simulink model "VU_testBtTxRx"  (Simulink 7.5)
settings: Solver=FixedStepDiscrete  SolverMode=SingleTasking  StartTime=0.0  StopTime=inf  FixedStep=0.1  RelTol=1e-3
libraries: lego_nxt_lib x5
settings Model: Creator=jpeytonj  LastModifiedBy=jpeytonj
settings RTWCC: SystemTargetFile=lrt.tlc  GenCodeOnly=on  TemplateMakefile=lrt_ecrobot.tmf  Description=Lego NXT Real-Time Target  ProcessScript=lrt_make_rtw_hook
settings STFCustomTargetCC: ModelReferenceCompliant=off  GeneratePreprocessorConditionals=Disable all  MatFileLogging=on  SystemTargetFile=lrt.tlc
settings GRTTargetCC: ModelReferenceCompliant=off  ParMdlRefBuildCompliant=off  CompOptLevelCompliant=off  ExtModeMexFile=noextcomm
settings CustomProperty: DataType=RTWOptions_EnumType_C__RTtools_VU-LRT_lrt_1codeGenType  Value=Integer-only
settings EnumStrPairs: String=Integer-only

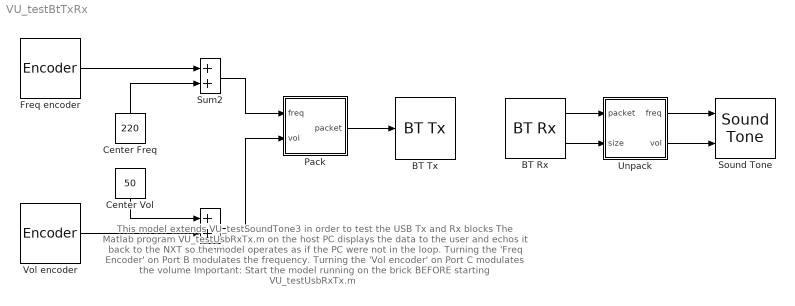
== system VU_testBtTxRx ==
  note: This model extends VU_testSoundTone3 in order to test the USB Tx and Rx blocks
      | The Matlab program VU_testUsbRxTx.m on the host PC displays the data to the user
      | and echos it back to the NXT so the model operates as if the PC were not in the loop.
      | Turning the 'Freq Encoder' on Port B modulates the frequency.
      | Turning the 'Vol encoder' on Port C modulates the volume
      |
      | Important:  Start the model running on the brick BEFORE starting VU_testUsbRxTx.m
  BT Rx : lego_nxt_lib/BT Rx  init_y0=zeros(32,1,'uint8')  mos=Slave  ip=0  st=0.1
  BT Tx : lego_nxt_lib/BT Tx  mos=Slave  ip=0
  Center Freq : Constant  Value=220  OutDataType=fixdt(1, 16)  OutScaling=2^0
  Center Vol : Constant  Value=50  OutDataType=fixdt(1, 16)  OutScaling=2^0
  Freq encoder : lego_nxt_lib/Encoder  port=Port B  st=0.1
  Pack : Stateflow chart  TreatAsAtomicUnit=on
  Sound Tone : lego_nxt_lib/Sound Tone  SystemSampleTime=-1  freqsrc=External  freq=220  volsrc=External  vol=70
  Sum1 : Sum  OutDataTypeMode=uint8  OutDataType=fixdt(1, 16)  OutScaling=2^0  OutDataTypeStr=uint8
  Sum2 : Sum  OutDataTypeMode=uint32  OutDataType=fixdt(1, 16)  OutScaling=2^0  OutDataTypeStr=uint32
  Unpack : Stateflow chart  TreatAsAtomicUnit=on
  Vol encoder : lego_nxt_lib/Encoder  port=Port C  st=0.1
  wires:
  Freq encoder/1 -> Sum2/1
  Center Freq/1 -> Sum2/2
  Vol encoder/1 -> Sum1/2
  Center Vol/1 -> Sum1/1
  BT Rx/1 -> Unpack/1(packet)
  BT Rx/2 -> Unpack/2(size)
  Unpack/1(freq) -> Sound Tone/1
  Sum2/1 -> Pack/1(freq)
  Sum1/1 -> Pack/2(vol)
  Pack/1(packet) -> BT Tx/1
  Unpack/2(vol) -> Sound Tone/2

== matlab function Pack ==
  data: freq input double; packet output double; vol input double
function packet = pack(freq,vol)

%First define the size of the packet
%using nullcopy to avoid generating unnecessary code
%uint32(freq)=4Bytes;  uint8(vol)=1Byte
packet= eml.nullcopy(zeros(5,1,'uint8'));

%Now construct the packet
packet= [typecast(freq,'uint8') typecast(vol,'uint8')]';

== matlab function Unpack ==
  data: packet input uint8; freq output double; size input uint8; vol output double
function [freq,vol] = unpack(packet,size)
% The parameter size defines the length of valid data
% within a  fixed size packet of 64 bytes

%Had to define input data types and sizes in Model Explorer to get this to work
%Would be nice if the Rx block defined these so that this block would simply inherit
%packet= eml.nullcopy(zeros(64,1,'uint8'));

%Simply deconstruct the packet
freq = typecast(packet(1:4),'uint32');
vol = uint8(packet(5));

if size~=5, freq = uint32(800); end;
